simulink model "Studio8_1"  (R2017b)
settings: Solver=ode45  StartTime=0.  StopTime=40  FixedStep=0.2  MaxStep=0.05  RelTol=1e-8  AbsTol=1e-8  EnableMultiTasking=on
settings Model: ExtModeTrigMode=oneshot  ExtModeArmWhenConnect=off  Creator=LEVIENKL  LastModifiedBy=carlislt
settings DataIOCC: SaveFormat=Array  SignalLoggingSaveFormat=ModelDataLogs  SaveOutput=off  SaveTime=off  SignalLoggingName=sigsOut
settings OptimizationCC: BlockReduction=off  BooleanDataType=off  ExpressionDepthLimit=2147483647  InitFltsAndDblsToZero=on  LifeSpan=inf
settings DebuggingCC: SaveWithParameterizedLinksMsg=none  UnderspecifiedInitializationDetection=Classic  MergeDetectMultiDrivingBlocksExec=none  SignalResolutionControl=TryResolveAllWithWarning  MultiTaskDSMMsg=warning  MultiTaskCondExecSysMsg=none  FcnCallInpInsideContextMsg=warning  AllowSymbolicDim=off  StateNameClashWarn=warning  SFUnexpectedBacktrackingDiag=warning  SFNoUnconditionalDefaultTransitionDiag=warning  SFExecutionAtInitializationDiag=none
settings HardwareCC: ProdBitPerPointer=32  ProdBitPerSizeT=32  ProdBitPerPtrDiffT=32  ProdLargestAtomicFloat=None  ProdIntDivRoundTo=Undefined  ProdEndianess=Unspecified  ProdWordSize=32  ProdHWDeviceType=32-bit Generic  TargetUnknown=on
settings ModelReferenceCC: PropagateSignalLabelsOutOfModel=off
settings CodeAppCC: StateflowObjectComments=on
settings GRTTargetCC: TargetFcnLib=ansi_tfl_tmw.mat  TargetLangStandard=C89/C90 (ANSI)  GeneratePreprocessorConditionals=Disable all  CombineOutputUpdateFcns=off  GRTInterface=on
settings ConfigComp: CovMetricSettings=dw  CovHtmlReporting=on  CovSaveCumulativeToWorkspaceVar=on  CovSaveSingleToWorkspaceVar=on  CovExternalEMLEnable=off  CovSFcnEnable=off

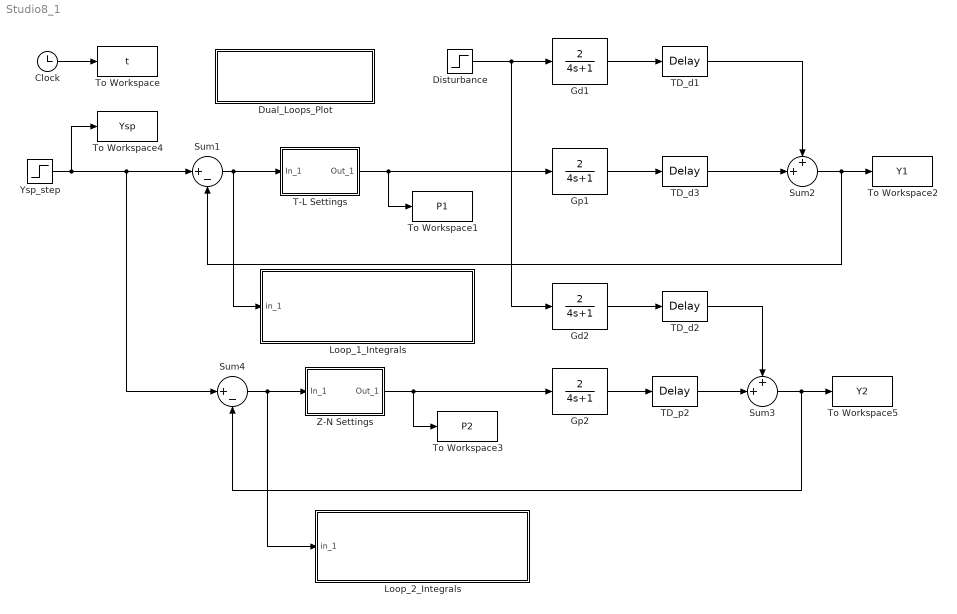
== system Studio8_1 ==
  Clock : Clock
  Disturbance : Step  Time=5  After=0  SampleTime=0
      settings: AttributesFormatString=%<Before> to %<After>\nat %<Time>
  Dual_Loops_Plot : Subsystem  mask(Daul Y,P Plots 2 Loops){}
      settings: OpenFcn=DualYP
      mask Help: This block two loops Y and P.
      mask Display: disp('After Simulation:\n Double Click for Plots\n (uses DualYP.m)')
  Gd1 : TransferFcn  Numerator=[2]  Denominator=[4 1]
  Gd2 : TransferFcn  Numerator=[2]  Denominator=[4 1]
  Gp1 : TransferFcn  Numerator=[2]  Denominator=[4 1]
  Gp2 : TransferFcn  Numerator=[2]  Denominator=[4 1]
  Loop_1_Integrals : Subsystem  mask(Integral Error (3) Evaluations){}
      settings: OpenFcn=I3errs1
      mask Help: This block calculates loop #1 IAE, ISE and ITAE.
      mask Display: disp('After Loop 1 Simulation:\n Double Click for IAE, ISE & ITAE\n (uses I3errs1.p)')
  Loop_2_Integrals : Subsystem  mask(3 Error evaluations){}
      settings: OpenFcn=I3errs2
      mask Help: This block calculates the IAE, the ISE and the ITAE.
      mask Display: disp('After Loop 2 Simulation:\n Double Click for IAE, ISE & ITAE\n (uses I3errs2.p)')
  Sum1 : Sum  Inputs=|+-  SaturateOnIntegerOverflow=on  InputSameDT=on  OutDataTypeStr=Inherit: Same as first input
  Sum2 : Sum  Inputs=++|  SaturateOnIntegerOverflow=on  InputSameDT=on  OutDataTypeStr=Inherit: Same as first input
  Sum3 : Sum  Inputs=++|  SaturateOnIntegerOverflow=on  InputSameDT=on  OutDataTypeStr=Inherit: Same as first input
  Sum4 : Sum  Inputs=|+-  SaturateOnIntegerOverflow=on  InputSameDT=on  OutDataTypeStr=Inherit: Same as first input
  T-L Settings : Subsystem  mask(PID(with alpha) Controller for ChE 461){Kc=0.5, tauIi=1/4, tauD=0, alpha=0.05}
      mask prompts: Kc "Controller gain:"; tauIi "Inv of Integral time constant (careful - this is I action ! ) :"; tauD "Derivative time constant:"; alpha "Alpha value (small)::"
      mask help:
      | Enter expressions for controller gain,
      | inverse of integral time constant
      | and derivative time constant and alpha.
      settings: AttributesFormatString=Kc = %<Kc>\n1/TauI = %<tauIi>\nTauD = %<tauD>
      mask Help: This block implements a PID controller where parameters are entered for the Controller Gain, inverse of Integral time constant and Derivative time constant.  Alpha here is equal to 0.01.   Unmask this block to see how it works. The derivative term is implemented using a true derivative block.
      mask Display: disp('PIDalpha')
  TD_d1 : TransportDelay
      settings: AttributesFormatString=Delay=%<DelayTime>
  TD_d2 : TransportDelay
      settings: AttributesFormatString=Delay=%<DelayTime>
  TD_d3 : TransportDelay
      settings: AttributesFormatString=Delay=%<DelayTime>
  TD_p2 : TransportDelay
      settings: AttributesFormatString=Delay=%<DelayTime>
  To Workspace : ToWorkspace  VariableName=t  SampleTime=-1
  To Workspace1 : ToWorkspace  VariableName=P1  SampleTime=-1
  To Workspace2 : ToWorkspace  VariableName=Y1  SampleTime=-1
  To Workspace3 : ToWorkspace  VariableName=P2  SampleTime=-1
  To Workspace4 : ToWorkspace  VariableName=Ysp  SampleTime=-1
  To Workspace5 : ToWorkspace  VariableName=Y2  SampleTime=-1
  Ysp_step : Step  Time=5  After=0  SampleTime=0
      settings: AttributesFormatString=%<Before> to %<After>\nat %<Time>
  Z-N Settings : Subsystem  mask(PID(with alpha) Controller for ChE 461){Kc=0.5, tauIi=1/4, tauD=0, alpha=0.05}
      mask prompts: Kc "Controller gain:"; tauIi "Inv of Integral time constant (careful - this is I action ! ) :"; tauD "Derivative time constant:"; alpha "Alpha value (small)::"
      mask help:
      | Enter expressions for controller gain,
      | inverse of integral time constant
      | and derivative time constant and alpha.
      settings: AttributesFormatString=Kc = %<Kc>\n1/TauI = %<tauIi>\nTauD = %<tauD>
      mask Help: This block implements a PID controller where parameters are entered for the Controller Gain, inverse of Integral time constant and Derivative time constant.  Alpha here is equal to 0.01.   Unmask this block to see how it works. The derivative term is implemented using a true derivative block.
      mask Display: disp('PIDalpha')
  wires:
  Clock/1 -> To Workspace/1
  Ysp_step/1 -> Sum4/1, Sum1/1, To Workspace4/1
  Sum2/1 -> Sum1/2, To Workspace2/1
  TD_d1/1 -> Sum2/1
  Sum1/1 -> Loop_1_Integrals/1(in_1), T-L Settings/1(In_1)
  T-L Settings/1(Out_1) -> Gp1/1, To Workspace1/1
  Gd1/1 -> TD_d1/1
  TD_d3/1 -> Sum2/2
  Sum3/1 -> Sum4/2, To Workspace5/1
  TD_d2/1 -> Sum3/1
  Z-N Settings/1(Out_1) -> Gp2/1, To Workspace3/1
  TD_p2/1 -> Sum3/2
  Disturbance/1 -> Gd2/1, Gd1/1
  Sum4/1 -> Loop_2_Integrals/1(in_1), Z-N Settings/1(In_1)
  Gp1/1 -> TD_d3/1
  Gp2/1 -> TD_p2/1
  Gd2/1 -> TD_d2/1

== system Studio8_1/Dual_Loops_Plot ==

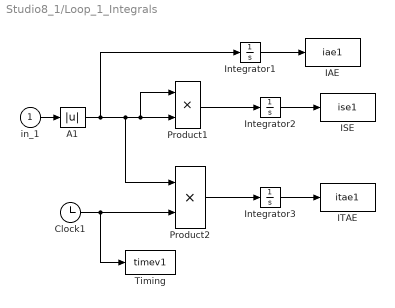
== system Studio8_1/Loop_1_Integrals ==
  in_1 : Inport
  A1 : Abs  ZeroCross=off  SaturateOnIntegerOverflow=on
  Clock1 : Clock
  IAE : ToWorkspace  VariableName=iae1
      settings: MaxDataPoints=20000
  ISE : ToWorkspace  VariableName=ise1
      settings: MaxDataPoints=20000
  ITAE : ToWorkspace  VariableName=itae1
      settings: MaxDataPoints=20000
  Integrator1 : Integrator
  Integrator2 : Integrator
  Integrator3 : Integrator
  Product1 : Product  SaturateOnIntegerOverflow=on  RndMeth=Zero  InputSameDT=on  OutDataTypeStr=Inherit: Same as first input
  Product2 : Product  SaturateOnIntegerOverflow=on  RndMeth=Zero  InputSameDT=on  OutDataTypeStr=Inherit: Same as first input
  Timing : ToWorkspace  VariableName=timev1
      settings: MaxDataPoints=20000
  wires:
  Integrator1/1 -> IAE/1
  Product1/1 -> Integrator2/1
  Clock1/1 -> Timing/1, Product2/2
  Integrator3/1 -> ITAE/1
  Integrator2/1 -> ISE/1
  Product2/1 -> Integrator3/1
  A1/1 -> Integrator1/1, Product2/1, Product1/1, Product1/2
  in_1/1 -> A1/1

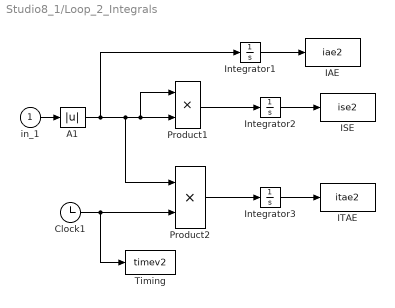
== system Studio8_1/Loop_2_Integrals ==
  in_1 : Inport
  A1 : Abs  ZeroCross=off  SaturateOnIntegerOverflow=on
  Clock1 : Clock
  IAE : ToWorkspace  VariableName=iae2
      settings: MaxDataPoints=20000
  ISE : ToWorkspace  VariableName=ise2
      settings: MaxDataPoints=20000
  ITAE : ToWorkspace  VariableName=itae2
      settings: MaxDataPoints=20000
  Integrator1 : Integrator
  Integrator2 : Integrator
  Integrator3 : Integrator
  Product1 : Product  SaturateOnIntegerOverflow=on  RndMeth=Zero  InputSameDT=on  OutDataTypeStr=Inherit: Same as first input
  Product2 : Product  SaturateOnIntegerOverflow=on  RndMeth=Zero  InputSameDT=on  OutDataTypeStr=Inherit: Same as first input
  Timing : ToWorkspace  VariableName=timev2
      settings: MaxDataPoints=20000
  wires:
  Integrator1/1 -> IAE/1
  Product1/1 -> Integrator2/1
  Clock1/1 -> Timing/1, Product2/2
  Integrator3/1 -> ITAE/1
  Integrator2/1 -> ISE/1
  Product2/1 -> Integrator3/1
  A1/1 -> Integrator1/1, Product2/1, Product1/1, Product1/2
  in_1/1 -> A1/1

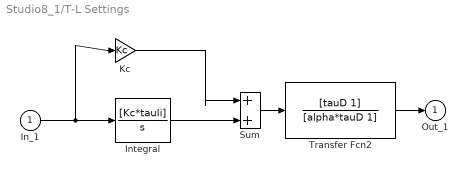
== system Studio8_1/T-L Settings ==
  In_1 : Inport
  Integral : TransferFcn  Numerator=[Kc*tauIi]  Denominator=[1 0]
  Kc : Gain  Gain=Kc  SaturateOnIntegerOverflow=on  OutDataTypeStr=Inherit: Same as input  ParamDataTypeStr=Inherit: Same as input
  Sum : Sum  SaturateOnIntegerOverflow=on  InputSameDT=on  OutDataTypeStr=Inherit: Same as first input
  Transfer Fcn2 : TransferFcn  Numerator=[tauD 1]  Denominator=[alpha*tauD 1]
  Out_1 : Outport
  wires:
  Transfer Fcn2/1 -> Out_1/1
  Sum/1 -> Transfer Fcn2/1
  In_1/1 -> Integral/1, Kc/1
  Integral/1 -> Sum/2
  Kc/1 -> Sum/1

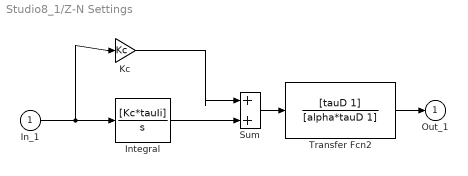
== system Studio8_1/Z-N Settings ==
  In_1 : Inport
  Integral : TransferFcn  Numerator=[Kc*tauIi]  Denominator=[1 0]
  Kc : Gain  Gain=Kc  SaturateOnIntegerOverflow=on  OutDataTypeStr=Inherit: Same as input  ParamDataTypeStr=Inherit: Same as input
  Sum : Sum  SaturateOnIntegerOverflow=on  InputSameDT=on  OutDataTypeStr=Inherit: Same as first input
  Transfer Fcn2 : TransferFcn  Numerator=[tauD 1]  Denominator=[alpha*tauD 1]
  Out_1 : Outport
  wires:
  Transfer Fcn2/1 -> Out_1/1
  Sum/1 -> Transfer Fcn2/1
  In_1/1 -> Integral/1, Kc/1
  Integral/1 -> Sum/2
  Kc/1 -> Sum/1
